simulink model "uz_endat_interface_2023a"  (R2023a)
settings: Solver=FixedStepDiscrete  StartTime=0.0  StopTime=1.3e-3  RelTol=1e-3
values from neighbouring files (symbols this model uses):
  binary_or_gray = false    [uz_endat_interface_init.m]
  bit_sum = endat_encoder_bit_width_multi_turn+endat_encoder_bit_width_single_turn+endat_encoder_number_of_CRC_bits    [uz_endat_interface_init.m]
  delay_first_clk_on_off = true    [uz_endat_interface_init.m]
  endat_clk_divider = 25    [uz_endat_interface_init.m]
  endat_encoder_bit_width_multi_turn = uint32(12)    [uz_endat_interface_init.m]
  endat_encoder_bit_width_single_turn = uint32(25)    [uz_endat_interface_init.m]
  endat_encoder_number_of_CRC_bits = uint32(0)    [uz_endat_interface_init.m]
  f_ADC = 20e3    (= 20000)    [uz_endat_interface_init.m]
  f_clock = 100e6    (= 100000000)    [uz_endat_interface_init.m]
  t_ADC = 1/f_ADC    (= 5e-05)    [uz_endat_interface_init.m]
  t_clock = 1/f_clock    (= 1e-08)    [uz_endat_interface_init.m]
undefined symbols (not defined in the file or in its folder): PLL
libraries: simulink x37, hdlsllib x21, simulink_extras x13, spsSampleandHoldLib x1
(part 1 of 2)
settings Model: DataTypeOverride=Off  Creator=micha  LastModifiedBy=micha
settings SolverCC: AlgebraicLoopSolver=TrustRegion
settings DataIOCC: LimitDataPoints=on  SaveOutput=off  SaveTime=off
settings OptimizationCC: BlockReduction=off  ConditionallyExecuteInputs=off  DefaultParameterBehavior=Inlined  InheritOutputTypeSmallerThanSingle=on  LifeSpan=inf
settings DebuggingCC: AlgebraicLoopMsg=error  SingleTaskRateTransMsg=error  UnconnectedInputMsg=warning  UnconnectedOutputMsg=warning  UnconnectedLineMsg=warning  AllowSymbolicDim=off  StrictBusMsg=ErrorOnBusTreatedAsVector  SFUnexpectedBacktrackingDiag=warning  SFNoUnconditionalDefaultTransitionDiag=warning  SFExecutionAtInitializationDiag=none  ArithmeticOperatorsInVariantConditions=warning
settings HardwareCC: ProdBitPerPointer=32  ProdBitPerSizeT=32  ProdBitPerPtrDiffT=32  ProdLargestAtomicFloat=None  ProdIntDivRoundTo=Undefined  ProdEndianess=Unspecified  ProdWordSize=32  ProdHWDeviceType=ASIC/FPGA->ASIC/FPGA  ProdEqTarget=off
settings ModelReferenceCC: EnableRefExpFcnMdlSchedulingChecks=on
settings SFSimCC: SimUseLocalCustomCode=off  CustomCodeUndefinedFunction=UseInterfaceOnly
settings RTWCC: RTWUseLocalCustomCode=off  DLArmComputeVersion=19.05
settings CodeAppCC: StateflowObjectComments=on
settings GRTTargetCC: TargetLangStandard=C89/C90 (ANSI)
settings ConfigComp: CovScope=ReferencedModels  CovMetricSettings=dw  CovSaveCumulativeToWorkspaceVar=on  CovSaveSingleToWorkspaceVar=on  CovExternalEMLEnable=off  CovSFcnEnable=off

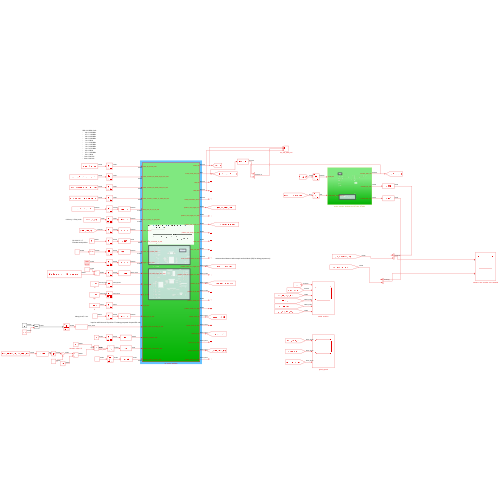
[thumbnail: Simulink's stored preview of the top-level diagram]
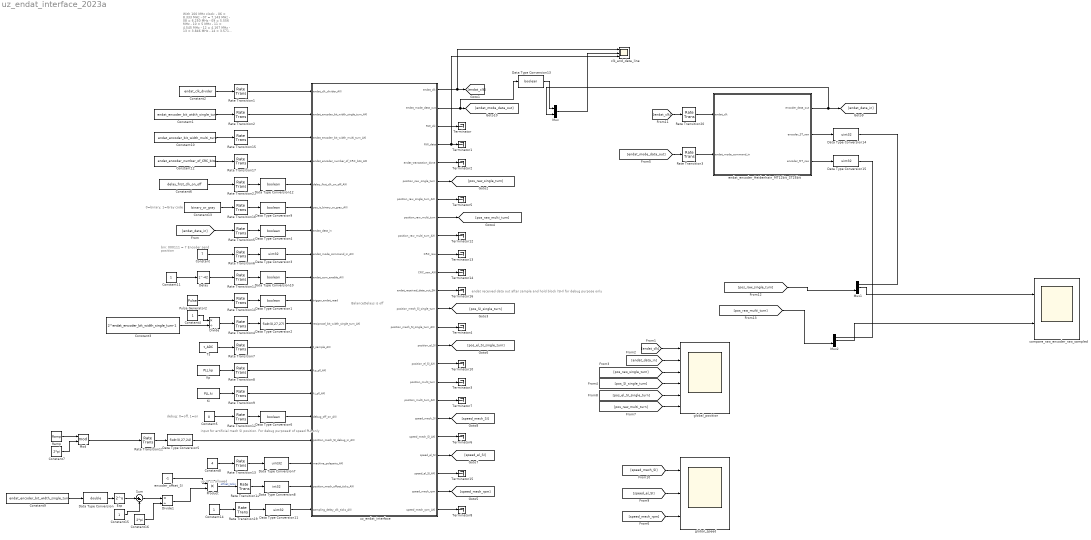
== system uz_endat_interface_2023a ==
  note: bin: 000111 = 7
      | Encoder send position
  note: input for artificial mech SI position. For debug purpose# of speed PLL only
  note: endat received data out after sample and hold block (SH) for debug purpose only
  note: up to 21 allowed
  note: debug: 0=off, 1=on
  note: BalanceDelays is off
  note: With 100 MHz clock:
      | -     06 = 8.333 MHz
      | -     07 = 7.143 MHz
      | -     08 = 6.250 MHz
      | -     09 = 5.556 MHz
      | -     10 = 5 MHz
      | -     11 = 4.545 MHz
      | -     12 = 4.167 MHz
      | -     13 = 3.846 MHz
      | -     14 = 3.571 MHz
      | -     25 = 2 MHz
      | -     27 = 1.852 MHz
      | -     50 = 1 MHz
      | -   100 = 500 kHz
      | -   200 = 250 kHz
  note: 0=binary, 1=Gray code
  Constant : Constant  Value=7  SampleTime=-1
  Constant1 : Constant  Value=endat_encoder_bit_width_single_turn  OutDataTypeStr=uint32  SampleTime=t_clock
  Constant10 : Constant  Value=endat_encoder_bit_width_multi_turn  OutDataTypeStr=uint32  SampleTime=t_clock
  Constant{4,11,14..15} (4 alike) : Constant  SampleTime=t_clock
  Constant12 : Constant  Value=endat_encoder_number_of_CRC_bits  OutDataTypeStr=uint32  SampleTime=t_clock
  Constant13 : Constant  Value=binary_or_gray  OutDataTypeStr=uint32  SampleTime=t_clock
  Constant16 : Constant  Value=2*pi  SampleTime=t_clock
  Constant2 : Constant  Value=endat_clk_divider  OutDataTypeStr=uint32  SampleTime=t_clock
  Constant3 : Constant  Value=2^endat_encoder_bit_width_single_turn-1  OutDataTypeStr=double  SampleTime=t_clock
  Constant5 : Constant  Value=0  SampleTime=t_clock
  Constant6 : Constant  Value=delay_first_clk_on_off  SampleTime=-1
  Constant7 : Constant  Value=2*pi  SampleTime=t_clock
  Constant8 : Constant  Value=4  SampleTime=t_clock
  Constant9 : Constant  Value=endat_encoder_bit_width_single_turn  OutDataTypeStr=uint32  SampleTime=t_clock
  Data Type Conversion : DataTypeConversion  OutDataTypeStr=double  SaturateOnIntegerOverflow=off  RndMeth=Floor
  Data Type Conversion{1,4,6,9..10,12..13} (7 alike) : DataTypeConversion  OutDataTypeStr=boolean  SaturateOnIntegerOverflow=off  RndMeth=Floor
  Data Type Conversion{3,7,11,14..15} (5 alike) : DataTypeConversion  OutDataTypeStr=uint32  SaturateOnIntegerOverflow=off  RndMeth=Floor
  Data Type Conversion2 : DataTypeConversion  OutDataTypeStr=fixdt(0,27,27)  SaturateOnIntegerOverflow=off  RndMeth=Floor
  Data Type Conversion5 : DataTypeConversion  OutDataTypeStr=fixdt(0,27,24)  SaturateOnIntegerOverflow=off  RndMeth=Floor
  Data Type Conversion8 : DataTypeConversion  OutDataTypeStr=int32  SaturateOnIntegerOverflow=off  RndMeth=Floor
  Delay : Delay  DelayLength=42
  Divide : Product  Inputs=*/
  Divide1 : Product  Inputs=*/
  Exp : Math  Operator=2^u
  Ki : Constant  Value=PLL.ki  OutDataTypeStr=fixdt(0,18,0)  SampleTime=-1
  Kp : Constant  Value=PLL.kp  OutDataTypeStr=fixdt(0,18,5)  SampleTime=-1
  Mod : Math  Operator=mod
  Mux : Mux  Inputs=2
  Mux1 : Mux  Inputs=2
  Mux2 : Mux  Inputs=2
  Product : Product
  Pulse Generator2 : DiscretePulseGenerator  Period=f_clock/f_ADC  PulseWidth=0.04*f_clock/f_ADC  PhaseDelay=250  SampleTime=t_clock
  Ramp : simulink/Sources/Ramp  slope=2*pi*100  start=7.5e-5  InitialOutput=0
  Rate Transition{1..21} (21 alike) : RateTransition  OutPortSampleTime=t_clock
  Sum : Sum  Inputs=|+-
  Terminator{,1..8,10,12..16} (15 alike) : Terminator
  Ts : Constant  Value=t_ADC  OutDataTypeStr=fixdt(0,18,24)  SampleTime=-1
  clk_and_data_line : Scope  NumInputPorts=3
  compare_raw_encoder_raw_sampled : Scope  NumInputPorts=2
  encoder_offset_SI : Constant  Value=-1  SampleTime=t_clock
  endat_encoder_Heidenhain_MT12bit_ST25bit : Subsystem
  global_position : Scope  NumInputPorts=6
  global_speed : Scope  NumInputPorts=3
  uz_endat_interface : Subsystem  TreatAsAtomicUnit=on
  wires:
  Rate Transition10/1 -> Data Type Conversion1/1
  Constant2/1 -> Rate Transition1/1
  Rate Transition1/1 -> uz_endat_interface/1(endat_clk_divider_AXI)
  Constant1/1 -> Rate Transition2/1
  Rate Transition2/1 -> uz_endat_interface/2(endat_encoder_bit_width_single_turn_AXI)
  [endat_data_in] -> Rate Transition5/1
  uz_endat_interface/1(endat_clk) -> clk_and_data_line/1, [endat_clk]
  uz_endat_interface/4(RW_data) -> clk_and_data_line/3, Terminator1/1
  uz_endat_interface/5(endat_transaction_done) -> Terminator2/1
  uz_endat_interface/3(RW_clk) -> Terminator/1
  Data Type Conversion1/1 -> uz_endat_interface/10(trigger_endat_read)
  uz_endat_interface/7(position_raw_single_turn_AXI) -> Terminator5/1
  Rate Transition5/1 -> Data Type Conversion4/1
  Data Type Conversion4/1 -> uz_endat_interface/7(endat_data_in)
  Constant3/1 -> Divide/2
  Rate Transition4/1 -> Data Type Conversion2/1
  Data Type Conversion2/1 -> uz_endat_interface/11(reciprocal_bit_width_single_turn_AXI)
  Constant4/1 -> Divide/1
  Divide/1 -> Rate Transition4/1
  uz_endat_interface/14(position_mech_SI_single_turn_AXI) -> Terminator4/1
  Ts/1 -> Rate Transition7/1
  Rate Transition7/1 -> uz_endat_interface/12(t_sample_AXI)
  Kp/1 -> Rate Transition8/1
  Rate Transition8/1 -> uz_endat_interface/13(kp_pll_AXI)
  Ki/1 -> Rate Transition9/1
  Rate Transition9/1 -> uz_endat_interface/14(ki_pll_AXI)
  uz_endat_interface/19(speed_mech_SI) -> [speed_mech_SI]
  uz_endat_interface/20(speed_mech_SI_AXI) -> Terminator6/1
  Rate Transition11/1 -> Data Type Conversion5/1
  Data Type Conversion5/1 -> uz_endat_interface/16(position_mech_SI_debug_in_AXI)
  Data Type Conversion6/1 -> uz_endat_interface/15(debug_off_on_AXI)
  Rate Transition12/1 -> Data Type Conversion6/1
  Constant5/1 -> Rate Transition12/1
  Mod/1 -> Rate Transition11/1
  Ramp/1 -> Mod/1
  Constant7/1 -> Mod/2
  uz_endat_interface/24(speed_mech_rpm_AXI) -> Terminator8/1
  Rate Transition13/1 -> Data Type Conversion7/1
  Data Type Conversion7/1 -> uz_endat_interface/17(machine_polepairs_AXI)
  Constant8/1 -> Rate Transition13/1
  Rate Transition14/1 -> Data Type Conversion8/1
  encoder_offset_SI/1 -> Product/1
  Data Type Conversion8/1 -> uz_endat_interface/18(position_mech_offset_ticks_AXI)
  uz_endat_interface/15(position_el_SI) -> [pos_el_SI_single_turn]
  uz_endat_interface/16(position_el_SI_AXI) -> Terminator10/1
  Rate Transition15/1 -> uz_endat_interface/3(endat_encoder_bit_width_multi_turn_AXI)
  Constant10/1 -> Rate Transition15/1
  Rate Transition16/1 -> Data Type Conversion9/1
  Constant13/1 -> Rate Transition16/1
  Data Type Conversion9/1 -> uz_endat_interface/6(pos_is_binary_or_gray_AXI)
  Rate Transition17/1 -> uz_endat_interface/4(endat_encoder_number_of_CRC_bits_AXI)
  Constant12/1 -> Rate Transition17/1
  Data Type Conversion10/1 -> uz_endat_interface/9(endat_com_enable_AXI)
  Rate Transition18/1 -> Data Type Conversion10/1
  Constant11/1 -> Delay/1
  uz_endat_interface/8(position_raw_multi_turn) -> [pos_raw_multi_turn]
  uz_endat_interface/9(position_raw_multi_turn_AXI) -> Terminator12/1
  uz_endat_interface/10(CRC_raw) -> Terminator13/1
  uz_endat_interface/11(CRC_raw_AXI) -> Terminator14/1
  uz_endat_interface/22(speed_el_SI_AXI) -> Terminator15/1
  uz_endat_interface/21(speed_el_SI) -> [speed_el_SI]
  [endat_clk] -> global_position/1
  [endat_data_in] -> global_position/2
  uz_endat_interface/6(position_raw_single_turn) -> [pos_raw_single_turn]
  [pos_raw_single_turn] -> global_position/3
  [pos_SI_single_turn] -> global_position/4
  uz_endat_interface/13(position_mech_SI_single_turn) -> [pos_SI_single_turn]
  uz_endat_interface/12(endat_received_data_out_SH) -> Terminator16/1
  uz_endat_interface/23(speed_mech_rpm) -> [speed_mech_rpm]
  Delay/1 -> Rate Transition18/1
  [speed_mech_rpm] -> global_speed/3
  [pos_raw_multi_turn] -> global_position/6
  [pos_el_SI_single_turn] -> global_position/5
  [speed_mech_SI] -> global_speed/1
  [speed_el_SI] -> global_speed/2
  Data Type Conversion11/1 -> uz_endat_interface/19(sampling_delay_clk_ticks_AXI)
  Rate Transition19/1 -> Data Type Conversion11/1
  Constant14/1 -> Rate Transition19/1
  [endat_clk] -> Rate Transition20/1
  Rate Transition20/1 -> endat_encoder_Heidenhain_MT12bit_ST25bit/1(endat_clk)
  endat_encoder_Heidenhain_MT12bit_ST25bit/1(encoder_data_out) -> Mux/2, [endat_data_in]
  uz_endat_interface/17(position_multi_turn) -> Terminator3/1
  uz_endat_interface/18(position_multi_turn_AXI) -> Terminator7/1
  Product/1 -> Rate Transition14/1  "offset_ticks"
  Constant9/1 -> Data Type Conversion/1
  Constant15/1 -> Sum/2
  Exp/1 -> Sum/1
  Sum/1 -> Divide1/1
  Constant16/1 -> Divide1/2
  Divide1/1 -> Product/2
  Data Type Conversion/1 -> Exp/1
  uz_endat_interface/2(endat_mode_data_out) -> Data Type Conversion13/1, [endat_mode_data_out]
  [endat_mode_data_out] -> Rate Transition3/1
  Rate Transition3/1 -> endat_encoder_Heidenhain_MT12bit_ST25bit/2(endat_mode_command_in)
  Data Type Conversion3/1 -> uz_endat_interface/8(endat_mode_command_in_AXI)
  Rate Transition6/1 -> Data Type Conversion3/1
  Constant/1 -> Rate Transition6/1
  Data Type Conversion12/1 -> uz_endat_interface/5(delay_first_clk_on_off_AXI)
  Constant6/1 -> Rate Transition21/1
  Rate Transition21/1 -> Data Type Conversion12/1
  Mux/1 -> clk_and_data_line/2
  Data Type Conversion13/1 -> Mux/1
  Pulse Generator2/1 -> Rate Transition10/1
  endat_encoder_Heidenhain_MT12bit_ST25bit/2(encoder_ST_raw) -> Data Type Conversion14/1
  endat_encoder_Heidenhain_MT12bit_ST25bit/3(encoder_MT_raw) -> Data Type Conversion15/1
  [pos_raw_single_turn] -> Mux1/2
  [pos_raw_multi_turn] -> Mux2/2
  Mux1/1 -> compare_raw_encoder_raw_sampled/1
  Mux2/1 -> compare_raw_encoder_raw_sampled/2
  Data Type Conversion14/1 -> Mux1/1
  Data Type Conversion15/1 -> Mux2/1

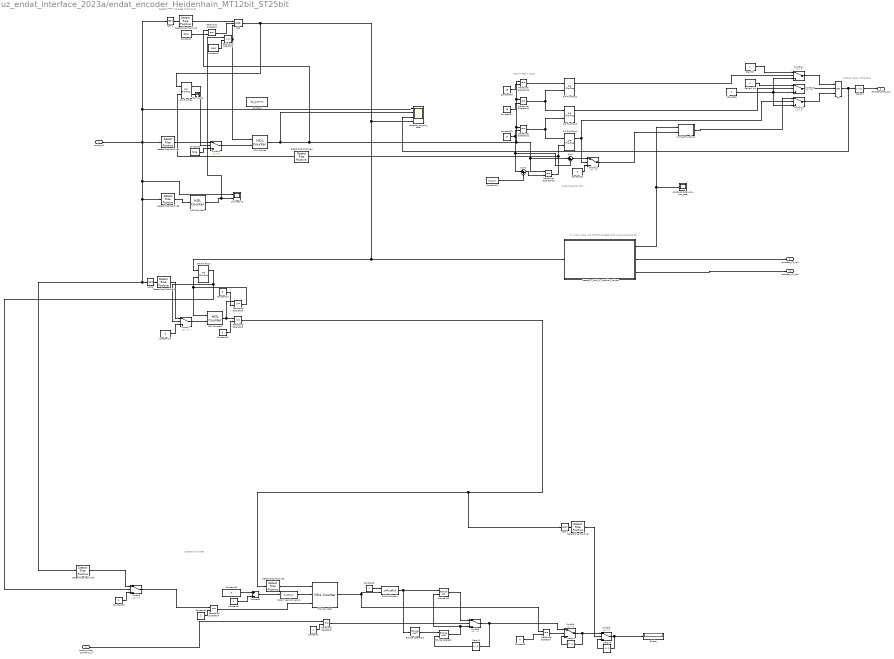
== system uz_endat_interface_2023a/endat_encoder_Heidenhain_MT12bit_ST25bit ==
  note: extend here for CRC
      | .
      | .
      | .
      | .
  note: fix output value with first falling edge of clk input to the encoder
  note: start bit after n clocks
  note: arbitrary delay of the data
  note: Detect first falling edge of the clock
  note: bitset and bit clear
  endat_clk : Inport
  endat_mode_command_in : Inport  Port=2
  AND : Logic  Inputs=3  IconShape=distinctive  AllPortsSameDT=off  OutDataTypeStr=boolean
  Bitwise Operator : simulink/Logic and Bit Operations/Bitwise Operator  logicop=AND  UseBitMask=off  NumInputPorts=2  BitMask=bin2dec('11011001')  BitMaskRealWorld=Stored Integer
  Bitwise Operator1 : simulink/Logic and Bit Operations/Bitwise Operator  logicop=NOT  UseBitMask=off  BitMask=bin2dec('11011001')  BitMaskRealWorld=Stored Integer
  Bitwise OR : simulink/Logic and Bit Operations/Bitwise Operator  logicop=OR  UseBitMask=off  NumInputPorts=2  BitMask=bin2dec('11011001')  BitMaskRealWorld=Stored Integer
      settings: LibrarySourceBlock=|
      | simulink/Quick Insert/Logic and Bit
      | Operations/Bitwise OR
  Constant : Constant  Value=bit_sum+1  SampleTime=t_clock
  Constant1 : Constant  Value=1000  OutDataTypeStr=uint32  SampleTime=t_clock
  Constant10 : Constant  Value=6  OutDataTypeStr=uint32  SampleTime=-1
  Constant11 : Constant  Value=3  OutDataTypeStr=uint32  SampleTime=-1
  Constant12 : Constant  Value=9  OutDataTypeStr=uint32  SampleTime=-1
  Constant13 : Constant  Value=0  OutDataTypeStr=boolean  SampleTime=t_clock
  Constant19 : Constant  Value=0  OutDataTypeStr=boolean  SampleTime=t_clock
  Constant2 : Constant  Value=false  SampleTime=t_clock
  Constant20 : Constant  Value=15  OutDataTypeStr=uint32  SampleTime=-1
  Constant21 : Constant  Value=16  OutDataTypeStr=uint32  SampleTime=-1
  Constant22 : Constant  Value=0  OutDataTypeStr=uint32  SampleTime=t_clock
  Constant23 : Constant  Value=17  OutDataTypeStr=uint32  SampleTime=-1
  Constant24 : Constant  Value=bit_sum  OutDataTypeStr=uint32  SampleTime=-1
  Constant3 : Constant  Value=false  SampleTime=t_clock
  Constant4 : Constant  OutDataTypeStr=boolean  SampleTime=t_clock
  Constant6 : Constant  OutDataTypeStr=uint64  SampleTime=t_clock
  Constant7 : Constant  OutDataTypeStr=boolean  SampleTime=t_clock
  Constant8 : Constant  Value=0  OutDataTypeStr=uint64  SampleTime=-1
  Constant9 : Constant  OutDataTypeStr=uint32  SampleTime=t_clock
  Data Type Conversion : DataTypeConversion  OutMin=0  OutMax=63  OutDataTypeStr=fixdt(0,6)  SaturateOnIntegerOverflow=off  RndMeth=Floor
  Delay1 : Delay  DelayLength=17  SampleTime=t_clock
  Delay5 : Delay  DelayLength=1
  Delay8 : Delay  DelayLength=1
  Delay9 : Delay  DelayLength=1  InitialCondition=0
  Detect Rise Positive{1..8} (8 alike) : simulink/Logic and Bit Operations/Detect Rise Positive  vinit=0  OutDataTypeStr=boolean
  Display : Display
  Fehler1 bit : Constant  Value=0  OutDataTypeStr=boolean  SampleTime=t_clock
  HDL Counter : hdlsllib/Sources/HDL Counter  CountType=Free running  CountInit=0  CountStep=1  CountMax=71  CountFromType=Initial value  CountFrom=0  CountResetPort=on  CountLoadPort=off  CountEnbPort=on  CountDirPort=off  CountHitOutputPort=off  CountDataType=Unsigned  CountWordLen=8  CountFracLen=0  CountSampTime=t_clock
  HDL Counter1 : hdlsllib/Sources/HDL Counter  CountType=Free running  CountInit=0  CountStep=1  CountMax=71  CountFromType=Initial value  CountFrom=0  CountResetPort=on  CountLoadPort=off  CountEnbPort=off  CountDirPort=off  CountHitOutputPort=off  CountDataType=Unsigned  CountWordLen=32  CountFracLen=0  CountSampTime=t_clock
  HDL Counter2 : hdlsllib/Sources/HDL Counter  CountType=Count limited  CountInit=1  CountStep=-1  CountMax=0  CountFromType=Initial value  CountFrom=1  CountResetPort=off  CountLoadPort=on  CountEnbPort=on  CountDirPort=off  CountHitOutputPort=off  CountDataType=Unsigned  CountWordLen=6  CountFracLen=0  CountSampTime=1
  HDL Counter4 : hdlsllib/Sources/HDL Counter  CountType=Free running  CountInit=0  CountStep=1  CountMax=4095  CountFromType=Initial value  CountFrom=0  CountResetPort=on  CountLoadPort=off  CountEnbPort=on  CountDirPort=off  CountHitOutputPort=off  CountDataType=Unsigned  CountWordLen=8  CountFracLen=0  CountSampTime=1
  MATLAB Function4 : MATLAB Function  TreatAsAtomicUnit=on
  NOT1 : Logic  Operator=NOT  IconShape=distinctive  AllPortsSameDT=off  OutDataTypeStr=boolean
  NOT3 : Logic  Operator=NOT  IconShape=distinctive  AllPortsSameDT=off  OutDataTypeStr=boolean
  NOT4 : Logic  Operator=NOT  IconShape=distinctive  AllPortsSameDT=off  OutDataTypeStr=boolean
  OR : Logic  Operator=OR  Inputs=3  IconShape=distinctive  AllPortsSameDT=off  OutDataTypeStr=boolean
  Relational Operator1 : RelationalOperator  OutDataTypeStr=boolean  RndMeth=Simplest  InputSameDT=off
  Relational Operator{2,4..5,7,10..13} (8 alike) : RelationalOperator  Operator===  OutDataTypeStr=boolean  RndMeth=Simplest  InputSameDT=off
  Relational Operator8 : RelationalOperator  OutDataTypeStr=boolean  RndMeth=Simplest  InputSameDT=off
  Relational Operator9 : RelationalOperator  OutDataTypeStr=boolean  RndMeth=Simplest  InputSameDT=off
  S-R Flip-Flop{,1..4} (5 alike) : simulink_extras/Flip Flops/S-R Flip-Flop  initial_condition=0
  Shift Arithmetic : ArithShift  BitShiftNumberSource=Input port  BitShiftNumber=8  BitShiftDirection=Left
      settings: InputPortMap=u0,p1
  Start bit : Constant  OutDataTypeStr=boolean  SampleTime=t_clock
  Subtract1 : Sum  Inputs=+-  OutDataTypeStr=uint32
  Sum : Sum  Inputs=|+-
  Sum2 : Sum  Inputs=|++
  Switch{1,5..13} (10 alike) : Switch  Criteria=u2 > Threshold  SaturateOnIntegerOverflow=off  InputSameDT=off
  Terminator : Terminator
  clk_inactive : Scope  NumInputPorts=2
  create_ST_and_MT_position_values : Subsystem
  encoder_cnt_and_data : Scope  NumInputPorts=4
  endat_encoder_raw_pos_data : Scope
  idle_state : Constant  Value=0  OutDataTypeStr=boolean  SampleTime=t_clock
  encoder_data_out : Outport
  encoder_ST_raw : Outport  Port=2
  encoder_MT_raw : Outport  Port=3
  wires:
  Relational Operator2/1 -> AND/2
  Constant2/1 -> Relational Operator2/2
  NOT1/1 -> Detect Rise Positive3/1
  Detect Rise Positive3/1 -> AND/1
  Delay1/1 -> encoder_data_out/1
  MATLAB Function4/1(y) -> Switch12/1
  Detect Rise Positive4/1 -> Switch7/1
  Data Type Conversion/1 -> HDL Counter2/2
  Delay8/1 -> Switch6/3
  Relational Operator7/1 -> Switch6/2
  Subtract1/1 -> Data Type Conversion/1  "pos"
  endat_mode_command_in/1 -> Relational Operator5/1
  Bitwise OR/1 -> Switch5/1
  Bitwise Operator/1 -> Switch5/3, Bitwise OR/2
  Constant9/1 -> Subtract1/2
  AND/1 -> S-R Flip-Flop/1, S-R Flip-Flop1/1, create_ST_and_MT_position_values/1(first_falling_edge_trigger), encoder_cnt_and_data/4
  Shift Arithmetic/1 -> Bitwise OR/1, Bitwise Operator1/1  "mask_set"
  Switch5/1 -> Switch6/1, Delay5/1
  Bitwise Operator1/1 -> Bitwise Operator/1  "mask_clear"
  Switch6/1 -> Delay8/1, Switch9/1
  Constant8/1 -> Relational Operator7/2
  Constant4/1 -> Relational Operator4/2
  Constant7/1 -> Relational Operator5/2
  Constant10/1 -> Subtract1/1  "bit_sum"
  Delay5/1 -> Bitwise Operator/2
  HDL Counter2/1 -> Shift Arithmetic/2, Relational Operator7/1  "pos"
  Relational Operator5/1 -> Switch5/2
  Detect Rise Positive5/1 -> HDL Counter2/1
  Relational Operator4/1 -> HDL Counter2/3
  Constant6/1 -> Shift Arithmetic/1
  Relational Operator8/1 -> Detect Rise Positive5/1, NOT4/1
  HDL Counter4/1 -> Relational Operator9/1, Relational Operator8/1  "MT_bin"
  Constant11/1 -> Relational Operator8/2
  Constant12/1 -> Relational Operator9/2
  Relational Operator9/1 -> HDL Counter4/1, S-R Flip-Flop1/2
  Switch7/1 -> HDL Counter4/2
  Constant13/1 -> Switch7/3
  NOT3/1 -> Detect Rise Positive4/1
  Detect Rise Positive6/1 -> Switch8/1
  Switch8/1 -> Relational Operator4/1
  Constant19/1 -> Switch8/3
  S-R Flip-Flop1/1 -> Switch8/2, Switch7/2
  Delay9/1 -> Switch9/3
  Switch9/1 -> Delay9/1, Display/1
  NOT4/1 -> Detect Rise Positive7/1
  Detect Rise Positive7/1 -> Switch9/2
  Constant20/1 -> Relational Operator10/2
  Relational Operator10/1 -> S-R Flip-Flop2/1
  S-R Flip-Flop2/1 -> Switch11/2
  Switch11/1 -> OR/1
  Constant21/1 -> Relational Operator11/2
  Relational Operator11/1 -> S-R Flip-Flop3/1, S-R Flip-Flop2/2
  Constant22/1 -> Switch10/3
  Start bit/1 -> Switch11/1
  Fehler1 bit/1 -> Switch13/1
  S-R Flip-Flop3/1 -> Switch13/2
  Constant23/1 -> Sum2/1, Sum/2, Relational Operator12/2
  Relational Operator12/1 -> S-R Flip-Flop4/1, S-R Flip-Flop3/2
  idle_state/1 -> Switch12/3, Switch13/3, Switch11/3
  OR/1 -> encoder_cnt_and_data/3, Delay1/1
  Switch12/1 -> OR/3
  Switch13/1 -> OR/2
  S-R Flip-Flop4/1 -> Switch12/2, Switch10/2
  Switch10/1 -> MATLAB Function4/2(cnt)
  Sum2/1 -> Relational Operator13/2
  Constant24/1 -> Sum2/2
  Sum/1 -> Switch10/1
  Relational Operator13/1 -> S-R Flip-Flop4/2, Detect Rise Positive2/1
  create_ST_and_MT_position_values/1(pos_data) -> MATLAB Function4/1(u), endat_encoder_raw_pos_data/1
  HDL Counter/1 -> encoder_cnt_and_data/2, Relational Operator10/1, Relational Operator11/1, Relational Operator12/1, Sum/1, Relational Operator13/1, Relational Operator2/1
  S-R Flip-Flop/1 -> Switch1/2
  Detect Rise Positive1/1 -> Switch1/1
  Switch1/1 -> HDL Counter/2
  Detect Rise Positive2/1 -> S-R Flip-Flop/2
  endat_clk/1 -> NOT1/1, encoder_cnt_and_data/1, clk_inactive/1, Detect Rise Positive8/1, Detect Rise Positive6/1, NOT3/1, Detect Rise Positive1/1
  Detect Rise Positive8/1 -> HDL Counter1/1
  HDL Counter1/1 -> Relational Operator1/1, clk_inactive/2
  Relational Operator1/1 -> AND/3, HDL Counter/1
  Constant1/1 -> Relational Operator1/2
  Constant3/1 -> Switch1/3
  S-R Flip-Flop/2 -> Terminator/1
  create_ST_and_MT_position_values/2(encoder_ST_raw) -> encoder_ST_raw/1
  create_ST_and_MT_position_values/3(encoder_MT_raw) -> encoder_MT_raw/1

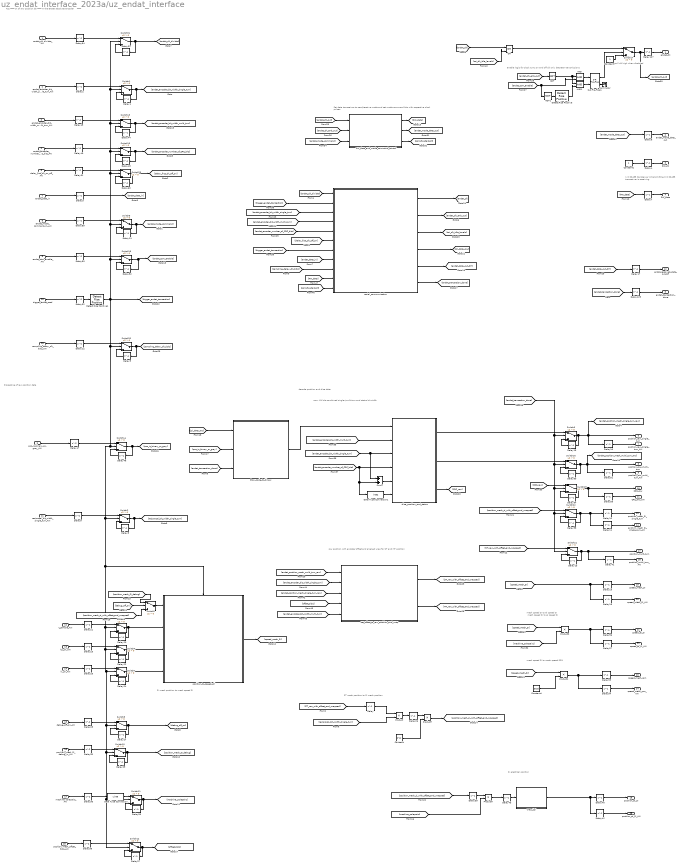
== system uz_endat_interface_2023a/uz_endat_interface ==
  note: Set data transceiver to send/receive mode and set mode command bits with respective clock pulses
  note: enable logic for clock: turns on and off clk only between transmissions
  note: pull clk high when disabled
  note: ST mech position to SI mech position
  note: 1 = RS485 transceiver is transmitting
      | 0 = RS485 transceiver is receiving
  note: Acquisition of raw position data from the EnDat absolute encoder
  note: SI mech position to mech speed SI
  note: mech speed SI to mech speed RPM
  note: SI electrical position
  note: mech speed SI to el speed SI
  note: max. 64 bits combined
      | single-/multi-turn and status bit width
  note: decode position and slice data
  note: mech speed SI to el speed SI
  note: Processing of raw position data
  note: raw position with encoder offset and aligned wrap for ST and MT position
  endat_clk_divider_AXI : Inport  OutDataTypeStr=uint32
  endat_encoder_bit_width_single_turn_AXI : Inport  Port=2  OutDataTypeStr=uint32
  endat_encoder_bit_width_multi_turn_AXI : Inport  Port=3  OutDataTypeStr=uint32
  endat_encoder_number_of_CRC_bits_AXI : Inport  Port=4  OutDataTypeStr=uint32
  delay_first_clk_on_off_AXI : Inport  Port=5  OutDataTypeStr=boolean
  pos_is_binary_or_gray_AXI : Inport  Port=6  OutDataTypeStr=boolean
  endat_data_in : Inport  Port=7
  endat_mode_command_in_AXI : Inport  Port=8  OutDataTypeStr=uint32
  endat_com_enable_AXI : Inport  Port=9  OutDataTypeStr=boolean
  trigger_endat_read : Inport  Port=10  OutDataTypeStr=boolean
  reciprocal_bit_width_single_turn_AXI : Inport  Port=11
  t_sample_AXI : Inport  Port=12
  kp_pll_AXI : Inport  Port=13
  ki_pll_AXI : Inport  Port=14
  debug_off_on_AXI : Inport  Port=15
  position_mech_SI_debug_in_AXI : Inport  Port=16
  machine_polepairs_AXI : Inport  Port=17
  position_mech_offset_ticks_AXI : Inport  Port=18
  sampling_delay_clk_ticks_AXI : Inport  Port=19  OutDataTypeStr=uint32
  AND : Logic  IconShape=distinctive  AllPortsSameDT=off  OutDataTypeStr=boolean
  AND1 : Logic  IconShape=distinctive  AllPortsSameDT=off  OutDataTypeStr=boolean
  Constant : Constant  Value=2*pi  OutDataTypeStr=fixdt(0,18,15)  SampleTime=t_clock
  Constant1 : Constant  OutDataTypeStr=boolean  SampleTime=t_clock
  Constant4 : Constant  Value=30/pi  OutDataTypeStr=fixdt(0,18,14)  SampleTime=-1
  Constant5 : Constant  OutDataTypeStr=boolean  SampleTime=t_clock
  Data Type Conversion : DataTypeConversion  OutDataTypeStr=uint8  SaturateOnIntegerOverflow=off  RndMeth=Floor
  Data Type Conversion1 : DataTypeConversion  OutDataTypeStr=int32  SaturateOnIntegerOverflow=off  RndMeth=Floor
  Delay{,14,20,22,24,26..27,29,37,60} (10 alike) : Delay  DelayLength=1  InitialCondition=0
  Delay1 : Delay  DelayLength=1  InitialCondition=endat_encoder_bit_width_single_turn
  Delay{4,6..8,10..11,16..19,33..34,39..40,42..43,56..58,129} (20 alike) : Delay  DelayLength=1
  Delay12 : Delay  InitialCondition=uint32(0)
  Delay127 : Delay  DelayLength=1  InitialCondition=1
  Delay{5,13,15,41,50..51,54..55} (8 alike) : Delay  DelayLength=1  InitialCondition=uint32(0)
  Delay{2..3,9,21,23,25,28,30,32,36,38,45,47,53,61,64} (16 alike) : Delay
  Delay31 : Delay  DelayLength=1  InitialCondition=endat_clk_divider
  Delay35 : Delay  DelayLength=1  InitialCondition=1
  Delay44 : Delay  DelayLength=1  InitialCondition=endat_encoder_bit_width_multi_turn
  Delay46 : Delay  DelayLength=1  InitialCondition=false
  Delay48 : Delay  DelayLength=1  InitialCondition=uint32(endat_encoder_number_of_CRC_bits)
  Delay49 : Delay  InitialCondition=uint32(0)
  Delay52 : Delay  DelayLength=1  InitialCondition=false
  Delay59 : Delay  InitialCondition=uint32(0)
  Detect Rise Positive : simulink/Logic and Bit Operations/Detect Rise Positive  vinit=0  OutDataTypeStr=boolean
  Detect Rise Positive1 : simulink/Logic and Bit Operations/Detect Rise Positive  vinit=0  OutDataTypeStr=boolean
  Gray_code_to_binary : Subsystem
  NOT : Logic  Operator=NOT  IconShape=distinctive  AllPortsSameDT=off  OutDataTypeStr=boolean
  NOT1 : Logic  Operator=NOT  IconShape=distinctive  AllPortsSameDT=off  OutDataTypeStr=boolean
  OR : Logic  Operator=OR  IconShape=distinctive  AllPortsSameDT=off  OutDataTypeStr=boolean
  Product : Product  OutDataTypeStr=fixdt(0,27,24)
  Product1 : Product  OutDataTypeStr=fixdt(1,27,12)
  Product2 : Product  OutDataTypeStr=fixdt(1,27,12)
  Product4 : Product  OutDataTypeStr=fixdt(0,27,20)
  Product7 : Product  OutDataTypeStr=fixdt(0,27,24)
  RW_data_and_mode_command_control : Subsystem
  S-R Flip-Flop1 : simulink_extras/Flip Flops/S-R Flip-Flop  initial_condition=0
  Sum2 : Sum  OutDataTypeStr=int32
  Switch{1..23,31} (24 alike) : Switch  Criteria=u2 > Threshold  SaturateOnIntegerOverflow=off  InputSameDT=off
  Terminator : Terminator
  position_to_speed_pll : Subsystem  TreatAsAtomicUnit=on
      settings: LibrarySourceBlock=|
      | hdlsllib/Ports &
      | Subsystems/Triggered
      | Subsystem
  serial_communication : Subsystem
  set_offset_to_raw_position_and_wrap : Subsystem
  slice_position_and_status : Subsystem
      settings: LibrarySourceBlock=|
      | hdlsllib/Ports &
      | Subsystems/Subsystem
  wrap_2pi : Subsystem
  endat_clk : Outport
  endat_mode_data_out : Outport  Port=2
  RW_clk : Outport  Port=3
  RW_data : Outport  Port=4
  endat_transaction_done : Outport  Port=5  OutDataTypeStr=boolean  LockScale=on
  position_raw_single_turn : Outport  Port=6  OutDataTypeStr=uint32  LockScale=on
  position_raw_single_turn_AXI : Outport  Port=7  OutDataTypeStr=uint32  LockScale=on
  position_raw_multi_turn : Outport  Port=8  OutDataTypeStr=uint32  LockScale=on
  position_raw_multi_turn_AXI : Outport  Port=9  OutDataTypeStr=uint32  LockScale=on
  CRC_raw : Outport  Port=10  OutDataTypeStr=uint32  LockScale=on
  CRC_raw_AXI : Outport  Port=11  OutDataTypeStr=uint32  LockScale=on
  endat_received_data_out_SH : Outport  Port=12
  position_mech_SI_single_turn : Outport  Port=13
  position_mech_SI_single_turn_AXI : Outport  Port=14
  position_el_SI : Outport  Port=15
  position_el_SI_AXI : Outport  Port=16
  position_multi_turn : Outport  Port=17  OutDataTypeStr=uint32  LockScale=on
  position_multi_turn_AXI : Outport  Port=18  OutDataTypeStr=uint32  LockScale=on
  speed_mech_SI : Outport  Port=19
  speed_mech_SI_AXI : Outport  Port=20
  speed_el_SI : Outport  Port=21
  speed_el_SI_AXI : Outport  Port=22
  speed_mech_rpm : Outport  Port=23
  speed_mech_rpm_AXI : Outport  Port=24
  wires:
  Delay129/1 -> endat_transaction_done/1
  trigger_endat_read/1 -> Delay32/1
  Delay32/1 -> Detect Rise Positive1/1
  Delay64/1 -> Switch31/1
  endat_clk_divider_AXI/1 -> Delay64/1
  Delay31/1 -> Switch31/3
  Switch31/1 -> Delay31/1, [endat_clk_divider]
  Switch1/1 -> Delay1/1, [endat_encoder_bit_width_single_turn]
  Delay1/1 -> Switch1/3
  endat_encoder_bit_width_single_turn_AXI/1 -> Delay2/1
  Delay2/1 -> Switch1/1
  endat_data_in/1 -> Delay3/1
  Delay127/1 -> endat_clk/1  "clk"
  Delay3/1 -> [endat_data_in]
  Switch6/1 -> [endat_position_mech_single_turn_raw], position_raw_single_turn/1, Delay16/1, Delay15/1
  Delay4/1 -> RW_clk/1
  Delay7/1 -> RW_data/1
  Constant1/1 -> Delay4/1
  [RW_data] -> Delay7/1
  Switch2/1 -> Delay8/1, [reciprocal_bit_width_single_turn]
  Delay9/1 -> Switch2/1
  Delay8/1 -> Switch2/3
  Delay10/1 -> position_mech_SI_single_turn/1
  Delay11/1 -> position_mech_SI_single_turn_AXI/1
  [ST_raw_with_offset_and_wrapped] -> Delay/1
  Delay15/1 -> Switch6/3
  Delay16/1 -> position_raw_single_turn_AXI/1
  Delay17/1 -> endat_received_data_out_SH/1
  reciprocal_bit_width_single_turn_AXI/1 -> Delay9/1
  Product/1 -> Delay26/1
  [position_mech_si_with_offset_and_wrapped] -> Switch9/3
  position_to_speed_pll/1(speed_mech_SI) -> [speed_mech_SI]
  [speed_mech_SI] -> Delay18/1, Delay19/1
  Delay19/1 -> speed_mech_SI/1
  Delay18/1 -> speed_mech_SI_AXI/1
  Delay20/1 -> Switch3/3
  Delay21/1 -> Switch3/1
  Switch3/1 -> position_to_speed_pll/2(t_sample), Delay20/1
  Switch4/1 -> position_to_speed_pll/3(kp_pll), Delay22/1
  Delay23/1 -> Switch4/1
  Delay22/1 -> Switch4/3
  Switch7/1 -> position_to_speed_pll/4(ki_pll), Delay24/1
  Delay25/1 -> Switch7/1
  Delay24/1 -> Switch7/3
  t_sample_AXI/1 -> Delay21/1
  kp_pll_AXI/1 -> Delay23/1
  ki_pll_AXI/1 -> Delay25/1
  Delay/1 -> Product/1
  [reciprocal_bit_width_single_turn] -> Product/2
  Delay26/1 -> Product7/1
  Product7/1 -> [position_mech_si_with_offset_and_wrapped]
  Switch8/1 -> [debug_off_on], Delay27/1
  Delay28/1 -> Switch8/1
  Delay27/1 -> Switch8/3
  Switch9/1 -> position_to_speed_pll/1(position_mech_SI)
  Delay30/1 -> Switch10/1
  Delay29/1 -> Switch10/3
  Switch10/1 -> [position_mech_SI_debug], Delay29/1
  [debug_off_on] -> Switch9/2
  debug_off_on_AXI/1 -> Delay28/1
  position_mech_SI_debug_in_AXI/1 -> Delay30/1
  [position_mech_SI_debug] -> Switch9/1
  Constant4/1 -> Product1/2
  [speed_mech_SI] -> Product1/1
  Product1/1 -> Delay33/1, Delay34/1
  Delay33/1 -> speed_mech_rpm/1
  Delay34/1 -> speed_mech_rpm_AXI/1
  Delay35/1 -> Switch11/3
  machine_polepairs_AXI/1 -> Delay36/1
  Delay36/1 -> Data Type Conversion/1
  Switch11/1 -> [machine_polepairs], Delay35/1
  Data Type Conversion/1 -> Switch11/1
  Detect Rise Positive1/1 -> [trigger_endat_transaction], Switch18/2, Switch5/2, Switch23/2, Switch13/2, Switch31/2, Switch1/2, Switch15/2, Switch20/2, Switch2/2, position_to_speed_pll/Trigger, Switch3/2, Switch4/2, Switch12/2, Switch11/2, Switch10/2, Switch8/2, Switch7/2, Switch14/2  "trigger_ssi"
  position_mech_offset_ticks_AXI/1 -> Delay38/1
  Switch12/1 -> [offset_ticks], Delay37/1
  Delay38/1 -> Switch12/1
  Delay37/1 -> Switch12/3
  [machine_polepairs] -> Product4/2
  wrap_2pi/1(output) -> Delay42/1, Delay40/1
  [position_mech_si_with_offset_and_wrapped] -> Delay39/1
  Product4/1 -> Delay43/1
  Switch22/1 -> Delay11/1, Delay10/1, Delay58/1
  Delay39/1 -> Product4/1
  Delay42/1 -> position_el_SI_AXI/1
  Delay40/1 -> position_el_SI/1
  Delay43/1 -> wrap_2pi/1(input)
  Delay44/1 -> Switch13/3
  Switch13/1 -> Delay44/1, [endat_encoder_bit_width_multi_turn]
  Delay45/1 -> Switch13/1
  endat_encoder_bit_width_multi_turn_AXI/1 -> Delay45/1
  pos_is_binary_or_gray_AXI/1 -> Delay47/1
  Delay46/1 -> Switch14/3
  Delay47/1 -> Switch14/1
  Switch14/1 -> Delay46/1, [pos_is_binary_or_gray]
  Delay49/1 -> Switch15/1
  Switch15/1 -> Delay48/1, [endat_encoder_number_of_CRC_bits]
  endat_encoder_number_of_CRC_bits_AXI/1 -> Delay49/1
  Delay48/1 -> Switch15/3
  Switch16/1 -> Delay50/1, position_raw_multi_turn/1, [endat_position_mech_multi_turn_raw], Delay51/1
  Delay51/1 -> position_raw_multi_turn_AXI/1
  Delay50/1 -> Switch16/3
  Constant/1 -> Product7/2
  OR/1 -> Switch17/1
  AND/1 -> S-R Flip-Flop1/1
  Constant5/1 -> Switch17/3
  Delay53/1 -> Switch18/1
  endat_com_enable_AXI/1 -> Delay53/1
  Switch18/1 -> [endat_com_enable], Delay52/1
  Delay52/1 -> Switch18/3
  [endat_com_enable] -> NOT1/1, AND/2
  NOT/1 -> AND1/1, AND/1
  [endat_clk_enb_out] -> NOT/1
  S-R Flip-Flop1/2 -> Terminator/1
  S-R Flip-Flop1/1 -> Switch17/2
  NOT1/1 -> Detect Rise Positive/1
  Detect Rise Positive/1 -> AND1/2
  Delay54/1 -> Switch19/3
  Switch19/1 -> CRC_raw/1, Delay55/1, Delay54/1
  Delay55/1 -> CRC_raw_AXI/1
  [endat_data_out_SH] -> Delay17/1
  [CRC_raw] -> Switch19/1
  AND1/1 -> S-R Flip-Flop1/2
  [speed_mech_SI] -> Product2/1
  Delay56/1 -> speed_el_SI/1
  Product2/1 -> Delay56/1, Delay57/1
  [machine_polepairs] -> Product2/2
  Delay57/1 -> speed_el_SI_AXI/1
  Data Type Conversion1/1 -> slice_position_and_status/6(shift_val_st)
  [endat_encoder_number_of_CRC_bits] -> Data Type Conversion1/1, Sum2/2, slice_position_and_status/4(bit_width_status)
  Sum2/1 -> slice_position_and_status/5(shift_val_mt)
  [endat_encoder_bit_width_single_turn] -> Sum2/1, slice_position_and_status/3(bit_width_st)
  [pos_is_binary_or_gray] -> Gray_code_to_binary/2(pos_is_binary_or_gray)
  slice_position_and_status/1(pos_raw_st) -> Switch6/1  "pos_bin_st"
  slice_position_and_status/2(pos_raw_mt) -> Switch16/1  "pos_bin_mt"
  slice_position_and_status/3(raw_CRC) -> [CRC_raw]  "status_raw"
  [endat_transaction_done] -> Delay129/1
  [ssi_clk_idle_levels] -> OR/2
  [trigger_endat_transaction] -> serial_communication/2(endat_clk_reset)
  [endat_encoder_bit_width_single_turn] -> serial_communication/3(bit_width_single_turn)
  [endat_encoder_bit_width_multi_turn] -> serial_communication/4(bit_width_multi_turn)
  [endat_encoder_number_of_CRC_bits] -> serial_communication/5(bit_width_CRC)
  [trigger_endat_transaction] -> serial_communication/7(trigger_endat)
  serial_communication/1(endat_clk) -> [endat_clk]
  serial_communication/2(endat_clk_enb_out) -> [endat_clk_enb_out]
  serial_communication/3(endat_clk_idle_levels) -> [ssi_clk_idle_levels]
  serial_communication/4(endat_data_raw) -> [ssi_data_raw]
  serial_communication/5(endat_data_SH) -> [endat_data_out_SH]
  serial_communication/6(endat_transaction_done) -> [endat_transaction_done]
  [endat_clk_divider] -> serial_communication/1(endat_clk_divider)
  [endat_clk] -> OR/1
  [endat_data_in] -> serial_communication/8(endat_data_in)
  Switch17/1 -> [endat_clk_out], Delay127/1
  [endat_transaction_done] -> Gray_code_to_binary/3(trigger)
  [ssi_data_raw] -> Gray_code_to_binary/1(ssi_data_raw)
  [endat_encoder_bit_width_multi_turn] -> slice_position_and_status/2(bit_width_mt)
  [sampling_delay_clk_ticks] -> serial_communication/9(sampling_delay_clk_ticks)
  Delay12/1 -> Switch20/1
  Delay5/1 -> Switch20/3
  sampling_delay_clk_ticks_AXI/1 -> Delay12/1
  Switch20/1 -> [sampling_delay_clk_ticks], Delay5/1
  Gray_code_to_binary/1(endat_pos_binary) -> slice_position_and_status/1(data)
  Switch21/1 -> Delay13/1, position_multi_turn/1, Delay41/1
  Delay13/1 -> Switch21/3
  Delay41/1 -> position_multi_turn_AXI/1
  [endat_transaction_done] -> Switch6/2, Switch16/2, Switch21/2, Switch22/2, Switch19/2
  [MT_raw_with_offset_and_wrapped] -> Switch21/1
  Delay58/1 -> Switch22/3
  [position_mech_si_with_offset_and_wrapped] -> Switch22/1
  [endat_position_mech_multi_turn_raw] -> set_offset_to_raw_position_and_wrap/1(mt_raw)  "mt_raw"
  [endat_encoder_bit_width_single_turn] -> set_offset_to_raw_position_and_wrap/2(n)  "n"
  [endat_position_mech_single_turn_raw] -> set_offset_to_raw_position_and_wrap/3(st_raw)  "st_raw"
  [offset_ticks] -> set_offset_to_raw_position_and_wrap/4(In4)
  [endat_encoder_bit_width_multi_turn] -> set_offset_to_raw_position_and_wrap/5(n1)  "n"
  set_offset_to_raw_position_and_wrap/1(st_raw_with_offset_and_wrapped) -> [ST_raw_with_offset_and_wrapped]
  set_offset_to_raw_position_and_wrap/2(mt_raw_with_offset_and_wrapped) -> [MT_raw_with_offset_and_wrapped]
  Delay6/1 -> endat_mode_data_out/1
  Delay59/1 -> Switch5/1
  Delay14/1 -> Switch5/3
  endat_mode_command_in_AXI/1 -> Delay59/1
  Switch5/1 -> Delay14/1, [endat_mode_command]
  Delay60/1 -> Switch23/3
  Delay61/1 -> Switch23/1
  delay_first_clk_on_off_AXI/1 -> Delay61/1
  Switch23/1 -> [delay_first_clk_off_on], Delay60/1
  [delay_first_clk_off_on] -> serial_communication/6(delay_first_clk_on_off)
  RW_data_and_mode_command_control/1(RW_data) -> [RW_data]
  [endat_clk_enb_out] -> RW_data_and_mode_command_control/2(endat_clk_enable)
  [endat_clk_out] -> RW_data_and_mode_command_control/1(endat_clk)
  [endat_mode_command] -> RW_data_and_mode_command_control/3(endat_mode_command)
  RW_data_and_mode_command_control/2(endat_mode_data_out) -> [endat_mode_data_out]
  [endat_mode_data_out] -> Delay6/1
  [RW_data] -> serial_communication/10(RW_data)
  RW_data_and_mode_command_control/3(poll_for_start_bit) -> [poll_for_start_bit]
  [poll_for_start_bit] -> serial_communication/11(poll_for_start_bit)

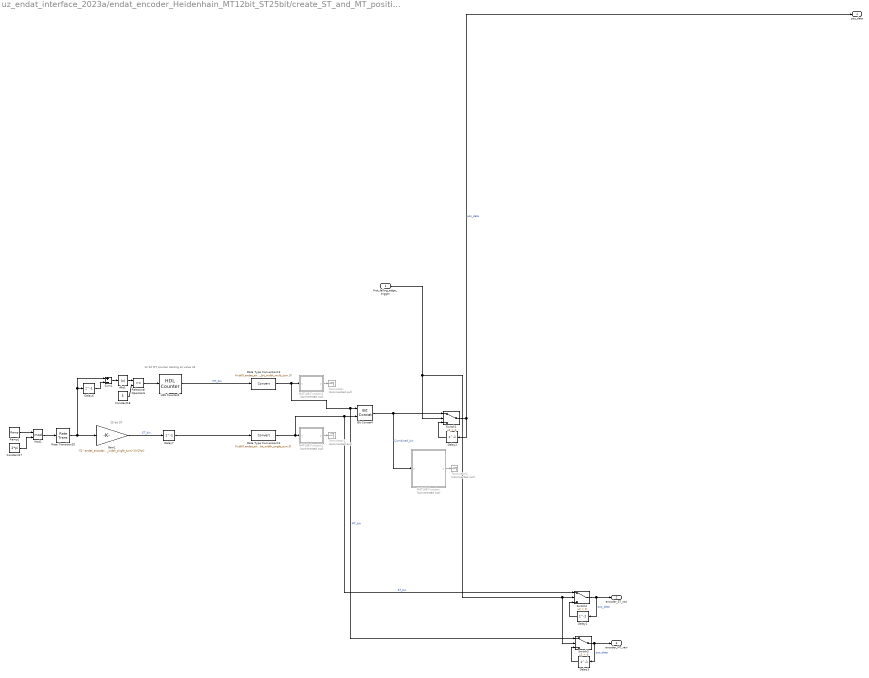
== system uz_endat_interface_2023a/endat_encoder_Heidenhain_MT12bit_ST25bit/create_ST_and_MT_position_values ==
  note: 12 bit MT counter starting at value 42
  note: 25 bit ST
  first_falling_edge_trigger : Inport
  Abs1 : Abs  SaturateOnIntegerOverflow=off
  Bit Concat4 : hdlsllib/Logic and Bit Operations/Bit Concat  numInputs=2
  Constant17 : Constant  Value=2*pi  SampleTime=t_clock
  Constant18 : Constant  Value=5  SampleTime=t_clock
  Data Type Conversion12 : DataTypeConversion  OutDataTypeStr=fixdt(0,endat_encoder_bit_width_single_turn,0)  SaturateOnIntegerOverflow=off  RndMeth=Floor
  Data Type Conversion13 : DataTypeConversion  OutDataTypeStr=fixdt(0,endat_encoder_bit_width_multi_turn,0)  SaturateOnIntegerOverflow=off  RndMeth=Floor
  Delay{1..3,6..7} (5 alike) : Delay  DelayLength=1
  Gain1 : Gain  Gain=((2^endat_encoder_bit_width_single_turn)-1)/(2*pi)  OutDataTypeStr=uint32
  HDL Counter3 : hdlsllib/Sources/HDL Counter  CountType=Count limited  CountInit=42  CountStep=1  CountMax=4095  CountFromType=Initial value  CountFrom=42  CountResetPort=off  CountLoadPort=off  CountEnbPort=on  CountDirPort=off  CountHitOutputPort=off  CountDataType=Unsigned  CountWordLen=12  CountFracLen=0  CountSampTime=1
  MATLAB Function : MATLAB Function  Commented=on  TreatAsAtomicUnit=on
  MATLAB Function1 : MATLAB Function  Commented=on  TreatAsAtomicUnit=on
  MATLAB Function2 : MATLAB Function  Commented=on  TreatAsAtomicUnit=on
  Mod1 : Math  Operator=mod
  Ramp1 : simulink/Sources/Ramp  slope=2*pi*50  start=0  InitialOutput=0
  Rate Transition20 : RateTransition  OutPortSampleTime=t_clock
  Relational Operator6 : RelationalOperator  OutDataTypeStr=boolean  RndMeth=Simplest  InputSameDT=off
  Sum1 : Sum  Inputs=+-
  Switch1 : Switch  Criteria=u2 > Threshold  SaturateOnIntegerOverflow=off  InputSameDT=off
  Switch2 : Switch  Criteria=u2 > Threshold  SaturateOnIntegerOverflow=off  InputSameDT=off
  Switch3 : Switch  Criteria=u2 > Threshold  SaturateOnIntegerOverflow=off  InputSameDT=off
  Terminator : Terminator  Commented=on
  Terminator1 : Terminator  Commented=on
  Terminator2 : Terminator  Commented=on
  pos_data : Outport
  encoder_ST_raw : Outport  Port=2
  encoder_MT_raw : Outport  Port=3
  wires:
  MATLAB Function2/1(y) -> Terminator/1
  Constant17/1 -> Mod1/2
  Data Type Conversion12/1 -> Switch2/1, Bit Concat4/2, MATLAB Function1/1(u)  "ST_bin"
  Constant18/1 -> Relational Operator6/2
  Delay7/1 -> Data Type Conversion12/1
  Rate Transition20/1 -> Sum1/1, Delay6/1, Gain1/1
  Switch1/1 -> pos_data/1, Delay2/1  "pos_data"
  HDL Counter3/1 -> Data Type Conversion13/1  "MT_bin"
  Bit Concat4/1 -> Switch1/1, MATLAB Function/1(u)  "Combined_bin"
  Ramp1/1 -> Mod1/1
  Data Type Conversion13/1 -> Switch3/1, Bit Concat4/1, MATLAB Function2/1(u)  "MT_bin"
  Relational Operator6/1 -> HDL Counter3/1
  Delay2/1 -> Switch1/3
  Delay6/1 -> Sum1/2
  Abs1/1 -> Relational Operator6/1
  Sum1/1 -> Abs1/1
  Gain1/1 -> Delay7/1  "ST_bin"
  Mod1/1 -> Rate Transition20/1
  MATLAB Function1/1(y) -> Terminator1/1
  MATLAB Function/1(y) -> Terminator2/1
  Switch2/1 -> encoder_ST_raw/1, Delay1/1  "pos_data"
  Delay1/1 -> Switch2/3
  first_falling_edge_trigger/1 -> Switch3/2, Switch2/2, Switch1/2
  Switch3/1 -> encoder_MT_raw/1, Delay3/1  "pos_data"
  Delay3/1 -> Switch3/3

== system uz_endat_interface_2023a/uz_endat_interface/Gray_code_to_binary ==
  ssi_data_raw : Inport
  pos_is_binary_or_gray : Inport  Port=2
  trigger : Inport  Port=3
  Delay : Delay  DelayLength=1
  Delay2 : Delay  DelayLength=101
  Delay6 : Delay  DelayLength=1
  Switch : Switch  Criteria=u2 > Threshold  SaturateOnIntegerOverflow=off  InputSameDT=off
  gray_to_bin : Subsystem
  endat_pos_binary : Outport
  wires:
  pos_is_binary_or_gray/1 -> Switch/2
  Switch/1 -> endat_pos_binary/1
  ssi_data_raw/1 -> Delay2/1, Delay/1
  Delay/1 -> gray_to_bin/1(gray)
  Delay2/1 -> Switch/3
  Delay6/1 -> Switch/1
  trigger/1 -> gray_to_bin/2(enb)
  gray_to_bin/1(binary_out) -> Delay6/1

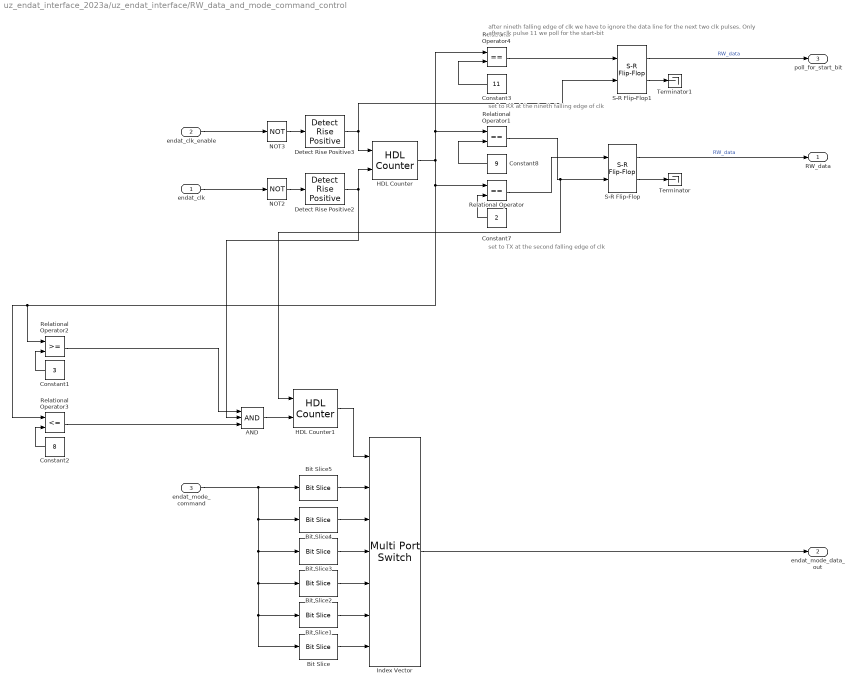
== system uz_endat_interface_2023a/uz_endat_interface/RW_data_and_mode_command_control ==
  note: set to TX at the second falling edge of clk
  note: set to RX at the nineth falling edge of clk
  note: after nineth falling edge of clk we have to ignore the data line for the next two clk pulses. Only after clk pulse 11 we poll for the start-bit
  endat_clk : Inport
  endat_clk_enable : Inport  Port=2
  endat_mode_command : Inport  Port=3
  AND : Logic  Inputs=3  IconShape=distinctive  AllPortsSameDT=off  OutDataTypeStr=boolean
  Bit Slice : hdlsllib/Logic and Bit Operations/Bit Slice  lidx=0  ridx=0
  Bit Slice1 : hdlsllib/Logic and Bit Operations/Bit Slice  lidx=1  ridx=1
  Bit Slice2 : hdlsllib/Logic and Bit Operations/Bit Slice  lidx=2  ridx=2
  Bit Slice3 : hdlsllib/Logic and Bit Operations/Bit Slice  lidx=3  ridx=3
  Bit Slice4 : hdlsllib/Logic and Bit Operations/Bit Slice  lidx=4  ridx=4
  Bit Slice5 : hdlsllib/Logic and Bit Operations/Bit Slice  lidx=5  ridx=5
  Constant1 : Constant  Value=3  OutDataTypeStr=uint8  SampleTime=-1
  Constant2 : Constant  Value=8  OutDataTypeStr=uint8  SampleTime=-1
  Constant3 : Constant  Value=11  OutDataTypeStr=uint8  SampleTime=-1
  Constant7 : Constant  Value=2  OutDataTypeStr=uint8  SampleTime=-1
  Constant8 : Constant  Value=9  OutDataTypeStr=uint8  SampleTime=-1
  Detect Rise Positive2 : simulink/Logic and Bit Operations/Detect Rise Positive  vinit=0  OutDataTypeStr=boolean
  Detect Rise Positive3 : simulink/Logic and Bit Operations/Detect Rise Positive  vinit=0  OutDataTypeStr=boolean
  HDL Counter : hdlsllib/Sources/HDL Counter  CountType=Free running  CountInit=0  CountStep=1  CountMax=25  CountFromType=Initial value  CountFrom=0  CountResetPort=on  CountLoadPort=off  CountEnbPort=on  CountDirPort=off  CountHitOutputPort=off  CountDataType=Unsigned  CountWordLen=8  CountFracLen=0  CountSampTime=1
  HDL Counter1 : hdlsllib/Sources/HDL Counter  CountType=Count limited  CountInit=0  CountStep=1  CountMax=5  CountFromType=Initial value  CountFrom=0  CountResetPort=on  CountLoadPort=off  CountEnbPort=on  CountDirPort=off  CountHitOutputPort=off  CountDataType=Unsigned  CountWordLen=8  CountFracLen=0  CountSampTime=1
  Index Vector : MultiPortSwitch  DataPortOrder=Zero-based contiguous  Inputs=6  zeroidx=on  SaturateOnIntegerOverflow=off  InputSameDT=off
  NOT2 : Logic  Operator=NOT  IconShape=distinctive  AllPortsSameDT=off  OutDataTypeStr=boolean
  NOT3 : Logic  Operator=NOT  IconShape=distinctive  AllPortsSameDT=off  OutDataTypeStr=boolean
  Relational Operator : RelationalOperator  Operator===  OutDataTypeStr=boolean  RndMeth=Simplest  InputSameDT=off
  Relational Operator1 : RelationalOperator  Operator===  OutDataTypeStr=boolean  RndMeth=Simplest  InputSameDT=off
  Relational Operator2 : RelationalOperator  OutDataTypeStr=boolean  RndMeth=Simplest  InputSameDT=off
  Relational Operator3 : RelationalOperator  Operator=<=  OutDataTypeStr=boolean  RndMeth=Simplest  InputSameDT=off
  Relational Operator4 : RelationalOperator  Operator===  OutDataTypeStr=boolean  RndMeth=Simplest  InputSameDT=off
  S-R Flip-Flop : simulink_extras/Flip Flops/S-R Flip-Flop  initial_condition=0
  S-R Flip-Flop1 : simulink_extras/Flip Flops/S-R Flip-Flop  initial_condition=0
  Terminator : Terminator
  Terminator1 : Terminator
  RW_data : Outport
  endat_mode_data_out : Outport  Port=2
  poll_for_start_bit : Outport  Port=3
  wires:
  Constant7/1 -> Relational Operator/2
  HDL Counter/1 -> Relational Operator2/1, Relational Operator3/1, Relational Operator/1, Relational Operator4/1, Relational Operator1/1
  endat_clk_enable/1 -> NOT3/1
  S-R Flip-Flop/2 -> Terminator/1
  Constant8/1 -> Relational Operator1/2
  NOT2/1 -> Detect Rise Positive2/1
  endat_clk/1 -> NOT2/1
  NOT3/1 -> Detect Rise Positive3/1
  S-R Flip-Flop/1 -> RW_data/1  "RW_data"
  Relational Operator/1 -> S-R Flip-Flop/1
  Detect Rise Positive3/1 -> HDL Counter/1, S-R Flip-Flop1/2
  Bit Slice/1 -> Index Vector/7
  Bit Slice3/1 -> Index Vector/4
  Bit Slice2/1 -> Index Vector/5
  Bit Slice1/1 -> Index Vector/6
  Bit Slice4/1 -> Index Vector/3
  Bit Slice5/1 -> Index Vector/2
  endat_mode_command/1 -> Bit Slice4/1, Bit Slice3/1, Bit Slice2/1, Bit Slice1/1, Bit Slice/1, Bit Slice5/1
  AND/1 -> HDL Counter1/2
  Constant1/1 -> Relational Operator2/2
  HDL Counter1/1 -> Index Vector/1
  Constant2/1 -> Relational Operator3/2
  Relational Operator1/1 -> HDL Counter1/1, S-R Flip-Flop/2
  Detect Rise Positive2/1 -> AND/2, HDL Counter/2
  Relational Operator2/1 -> AND/1
  Relational Operator3/1 -> AND/3
  Index Vector/1 -> endat_mode_data_out/1
  Constant3/1 -> Relational Operator4/2
  Relational Operator4/1 -> S-R Flip-Flop1/1
  S-R Flip-Flop1/1 -> poll_for_start_bit/1  "RW_data"
  S-R Flip-Flop1/2 -> Terminator1/1
